simulink model "Optimization_Model"  (R2020a)
settings: Solver=VariableStepAuto  StartTime=0.0  StopTime=23  FixedStep=0.002  RelTol=1e-3  EnableMultiTasking=on
undefined symbols (not defined in the file): shaveLevels
libraries: simulink x2
settings Model: ExtModeTrigDuration=10000  Creator=jeffm  LastModifiedBy=jeffm
settings SolverCC: PositivePriorityOrder=on
settings DataIOCC: ExternalInput=ts  LoadExternalInput=on  ReturnWorkspaceOutputsName=optimizationOut
settings OptimizationCC: LifeSpan=inf
settings DebuggingCC: ArithmeticOperatorsInVariantConditions=warning
settings SFSimCC: SimUseLocalCustomCode=off  CustomCodeUndefinedFunction=UseInterfaceOnly
settings RTWCC: Description=QUARC Win64 Target  SystemTargetFile=quarc_win64.tlc  TemplateMakefile=quarc_default_tmf  RTWUseLocalCustomCode=off
settings CodeAppCC: StateflowObjectComments=on
settings STFCustomTargetCC: TargetPreCompLibLocation=C:\PROGRA~3\QUARC\lib\2016a\win64\release  TargetLangStandard=C99 (ISO)  ConcurrentExecutionCompliant=on  GRTInterface=on  SystemTargetFile=quarc_win64.tlc
settings GRTTargetCC: TargetPreCompLibLocation=C:\PROGRA~3\QUARC\lib\2016a\win64\release  ParMdlRefBuildCompliant=off  CompOptLevelCompliant=off  CombineOutputUpdateFcns=off  MatFileLogging=off  CPPClassGenCompliant=off  GRTInterface=on  UseToolchainInfoCompliant=off  ExtMode=on  ExtModeMexFile=quarc_comm
settings ConfigComp: CovMetricSettings=dswe

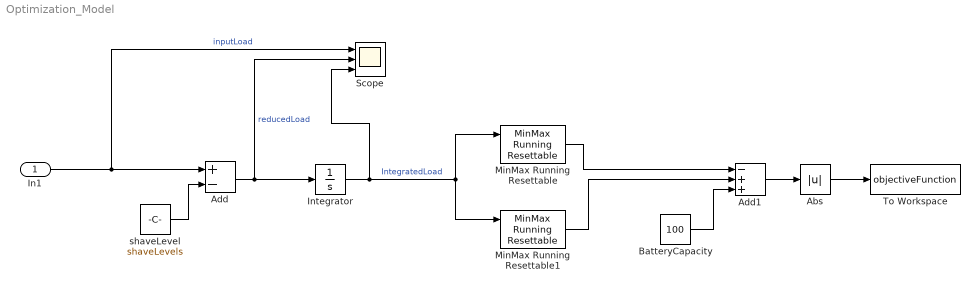
== system Optimization_Model ==
  In1 : Inport
  Abs : Abs
  Add : Sum  Inputs=+-
  Add1 : Sum  Inputs=-++
  BatteryCapacity : Constant  Value=100
  Integrator : Integrator
  MinMax Running Resettable : simulink/Math Operations/MinMax Running Resettable  Function=max  vinit=0
  MinMax Running Resettable1 : simulink/Math Operations/MinMax Running Resettable  Function=min  vinit=1000000
  Scope : Scope  NumInputPorts=3
  To Workspace : ToWorkspace  VariableName=objectiveFunction  SaveFormat=Timeseries  SampleTime=-1
  shaveLevel : Constant  Value=shaveLevels  VectorParams1D=off
  wires:
  shaveLevel/1 -> Add/2
  In1/1 -> Scope/1, Add/1  "inputLoad"
  Add/1 -> Integrator/1, Scope/2  "reducedLoad"
  Integrator/1 -> Scope/3, MinMax Running Resettable1/1, MinMax Running Resettable/1  "IntegratedLoad"
  MinMax Running Resettable/1 -> Add1/1
  MinMax Running Resettable1/1 -> Add1/2
  BatteryCapacity/1 -> Add1/3
  Add1/1 -> Abs/1
  Abs/1 -> To Workspace/1
